simulink model "sampleModel1708_1_sub"  (R2023a)
settings: Solver=VariableStepAuto  StartTime=0.0  StopTime=10.0  RelTol=1e-3
libraries: simulink x4, hdlsllib x3
settings Model: Creator=user1  LastModifiedBy=user1
settings OptimizationCC: BlockReduction=off  ConditionallyExecuteInputs=off

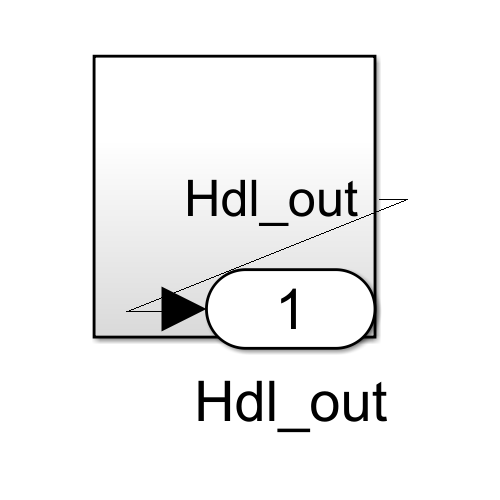
[thumbnail: Simulink's stored preview of the top-level diagram]
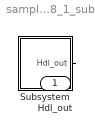
== system sampleModel1708_1_sub ==
  Subsystem : Subsystem
  Hdl_out : Outport  OutDataTypeStr=uint8
  wires:
  Subsystem/1(Hdl_out) -> Hdl_out/1

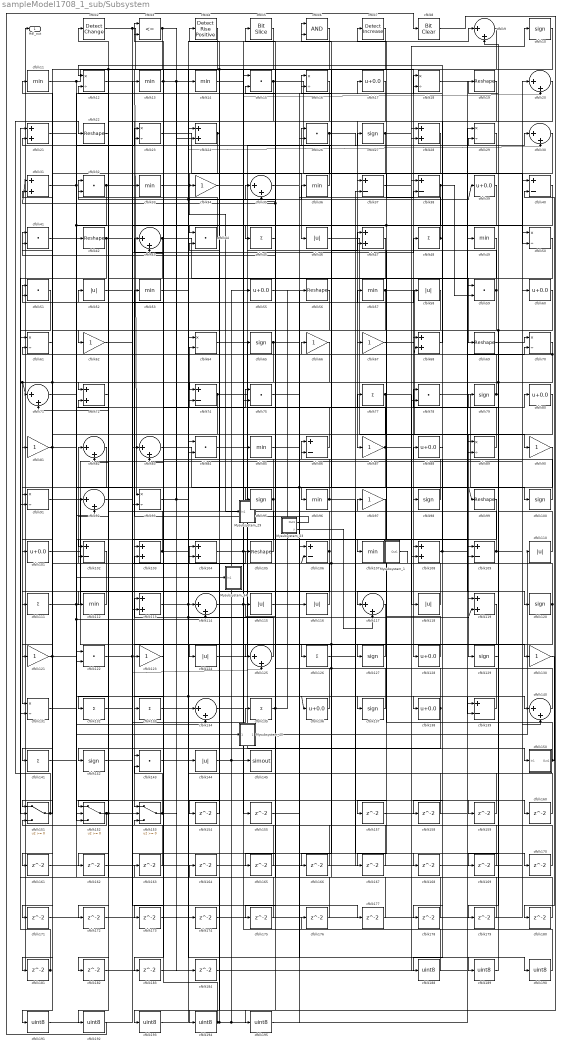
== system sampleModel1708_1_sub/Subsystem ==
  Mysubsystem_1 : Subsystem  TreatAsAtomicUnit=on  RTWFcnName=Mysubsystem_1
      settings: RTWFcnNameOpts=User specified  RTWFileNameOpts=Use function name
  Mysubsystem_23 : Subsystem  TreatAsAtomicUnit=on  RTWFcnName=Mysubsystem_23
      settings: RTWFcnNameOpts=User specified  RTWFileNameOpts=Use function name
  Mysubsystem_29 : Subsystem  TreatAsAtomicUnit=on  RTWFcnName=Mysubsystem_29
      settings: RTWFcnNameOpts=User specified  RTWFileNameOpts=Use function name
  Mysubsystem_34 : Subsystem  TreatAsAtomicUnit=on  RTWFcnName=Mysubsystem_34
      settings: RTWFcnNameOpts=User specified  RTWFileNameOpts=Use function name
  Mysubsystem_40 : Subsystem  TreatAsAtomicUnit=on  RTWFcnName=Mysubsystem_40
      settings: RTWFcnNameOpts=User specified  RTWFileNameOpts=Use function name
  cfblk{10,27,65,79,95,98,100,120,127,129,137,142} (12 alike) : Signum
  cfblk{17,39,55,60,80,88,101,128,136,138} (10 alike) : Bias  Bias=0.0  SaturateOnIntegerOverflow=off
  cfblk{37..38,40,74,86,102,106,109,139} (9 alike) : Sum  Inputs=+-  OutDataTypeStr=uint8
  cfblk{21,24,28,31,47,68,72,103..104,108,113,119} (12 alike) : Sum  OutDataTypeStr=uint8
  cfblk{19,22,42,56,69,99,105} (7 alike) : Reshape
  cfblk{11,13..14,33,36,49,53,57,85,96,107,112} (12 alike) : MinMax  OutDataTypeStr=uint8
  cfblk{46,52,58,110,115..116,118,124,144} (9 alike) : Abs  OutDataTypeStr=uint8  SaturateOnIntegerOverflow=off
  cfblk{45,48,77,111,126,132..133,135,141} (9 alike) : Sum  Inputs=+  OutDataTypeStr=uint8
  cfblk{9,20,30,35,43,71,82..83,92,114,117,125,134,140} (14 alike) : Sum  Inputs=|++  OutDataTypeStr=uint8
  cfblk{12,16,18,23,29,50,61,64,70,89,91,93,131} (13 alike) : Product  Inputs=*/  OutDataTypeStr=uint8  RndMeth=Zero  SaturateOnIntegerOverflow=on
  cfblk{34,62,66..67,81,87,90,97,121,123,130} (11 alike) : Gain  OutDataTypeStr=uint8
  cfblk{15,26,32,41,44,51,59,75,78,84,122,143} (12 alike) : DotProduct  OutDataTypeStr=uint8
  cfblk145 : ToWorkspace  VariableName=simout  SaveFormat=Timeseries  SampleTime=-1
  cfblk150 : Subsystem
      settings: LibrarySourceBlock=|
      | hdlsllib/Ports &
      | Subsystems/Subsystem
  cfblk151 : Switch  OutDataTypeStr=uint8  SaturateOnIntegerOverflow=off  InputSameDT=off
  cfblk152 : Switch  OutDataTypeStr=uint8  SaturateOnIntegerOverflow=off  InputSameDT=off
  cfblk153 : Switch  OutDataTypeStr=uint8  SaturateOnIntegerOverflow=off  InputSameDT=off
  cfblk{154..155,157..184} (30 alike) : Delay  SampleTime=1
  cfblk{188..195} (8 alike) : DataTypeConversion  OutDataTypeStr=uint8  SaturateOnIntegerOverflow=off  RndMeth=Floor
  cfblk2 : simulink/Logic and Bit Operations/Detect Change  vinit=0  OutDataTypeStr=uint8
      settings: LibrarySourceBlock=|
      | hdlsllib/Logic and Bit
      | Operations/Detect
      | Change
  cfblk3 : RelationalOperator  Operator=<=  OutDataTypeStr=boolean  InputSameDT=off
  cfblk4 : hdlsllib/Logic and Bit Operations/Detect Rise Positive  vinit=0  OutDataTypeStr=uint8
  cfblk5 : hdlsllib/Logic and Bit Operations/Bit Slice  lidx=7  ridx=0
  cfblk6 : Logic  AllPortsSameDT=off  OutDataTypeStr=boolean
  cfblk7 : simulink/Logic and Bit Operations/Detect Increase  vinit=0.0  OutDataTypeStr=uint8
      settings: LibrarySourceBlock=|
      | hdlsllib/Logic and Bit
      | Operations/Detect
      | Increase
  cfblk8 : simulink/Logic and Bit Operations/Bit Clear  iBit=0
      settings: LibrarySourceBlock=|
      | hdlsllib/Logic and Bit
      | Operations/Bit Clear
  Hdl_out : Outport  OutDataTypeStr=uint8
  wires:
  cfblk16/1 -> cfblk153/1
  cfblk26/1 -> cfblk29/2, cfblk34/1, Mysubsystem_29/1(In1)
  cfblk11/1 -> cfblk153/2, cfblk128/1
  cfblk17/1 -> cfblk87/1
  cfblk91/1 -> cfblk127/1
  cfblk65/1 -> cfblk30/1, cfblk131/1
  cfblk68/1 -> cfblk12/1
  cfblk57/1 -> cfblk83/2, cfblk90/1
  cfblk121/1 -> cfblk181/1, cfblk74/2
  cfblk10/1 -> cfblk74/1, cfblk93/1
  cfblk84/1 -> cfblk27/1
  cfblk95/1 -> cfblk152/3, cfblk4/1
  cfblk64/1 -> cfblk150/1(In1)
  cfblk106/1 -> cfblk122/2, cfblk43/1
  cfblk52/1 -> cfblk13/1
  cfblk24/1 -> cfblk191/1, cfblk44/1
  cfblk151/1 -> cfblk31/2, cfblk22/1
  cfblk53/1 -> cfblk136/1, cfblk144/1
  cfblk23/1 -> cfblk46/1
  cfblk4/1 -> cfblk123/1
  cfblk9/1 -> cfblk96/1
  cfblk98/1 -> cfblk86/1
  cfblk116/1 -> cfblk82/1
  cfblk124/1 -> cfblk36/1
  cfblk111/1 -> cfblk60/1, Mysubsystem_40/1(In1)
  cfblk105/1 -> cfblk2/1
  cfblk126/1 -> cfblk80/1
  cfblk46/1 -> cfblk129/1
  cfblk78/1 -> cfblk100/1
  cfblk123/1 -> cfblk23/1
  cfblk114/1 -> cfblk6/2, cfblk77/1
  cfblk81/1 -> cfblk41/1, cfblk93/2
  cfblk92/1 -> cfblk48/1
  cfblk29/1 -> cfblk142/1
  cfblk104/1 -> cfblk20/2, cfblk47/1
  cfblk28/1 -> cfblk67/1
  cfblk58/1 -> cfblk107/1
  cfblk137/1 -> cfblk31/1, cfblk32/1
  cfblk3/1 -> cfblk24/2, cfblk162/1, cfblk151/1
  cfblk79/1 -> cfblk9/2, cfblk61/2
  cfblk90/1 -> cfblk141/1
  cfblk56/1 -> cfblk143/1
  cfblk133/1 -> cfblk58/1
  cfblk30/1 -> cfblk68/1
  cfblk83/1 -> cfblk108/1
  cfblk42/1 -> cfblk108/2, cfblk131/2
  cfblk128/1 -> cfblk104/1
  cfblk50/1 -> cfblk103/1
  cfblk6/1 -> cfblk62/1
  cfblk74/1 -> cfblk183/1, cfblk138/1
  cfblk97/1 -> cfblk124/1
  cfblk117/1 -> cfblk166/1, cfblk165/1
  cfblk125/1 -> cfblk113/1
  cfblk70/1 -> cfblk68/2, cfblk169/1, cfblk91/2, cfblk81/1
  cfblk138/1 -> cfblk182/1, cfblk41/2, cfblk6/1
  cfblk39/1 -> cfblk117/1
  cfblk20/1 -> cfblk102/1
  cfblk66/1 -> cfblk101/1, cfblk71/1
  cfblk5/1 -> cfblk84/2
  cfblk127/1 -> cfblk125/1
  cfblk139/1 -> cfblk35/1
  cfblk67/1 -> cfblk98/1
  cfblk102/1 -> cfblk112/1
  cfblk61/1 -> cfblk11/1
  cfblk109/1 -> cfblk44/2, cfblk40/1
  cfblk21/1 -> cfblk50/2, cfblk42/1
  cfblk142/1 -> cfblk135/1
  cfblk48/1 -> cfblk7/1, cfblk18/1
  cfblk15/1 -> cfblk72/1, cfblk50/1
  cfblk69/1 -> cfblk70/1
  cfblk43/1 -> cfblk172/1, cfblk69/1
  cfblk153/1 -> cfblk184/1, cfblk143/2
  cfblk13/1 -> cfblk173/1, cfblk174/1, cfblk45/1
  cfblk112/1 -> cfblk111/1
  cfblk120/1 -> cfblk72/2, cfblk133/1
  cfblk51/1 -> cfblk151/2
  cfblk101/1 -> cfblk119/1
  cfblk113/1 -> cfblk126/1, cfblk9/1
  cfblk75/1 -> cfblk139/2, cfblk99/1
  cfblk87/1 -> cfblk109/2, cfblk121/1, cfblk3/1
  cfblk140/1 -> cfblk26/1
  cfblk150/1(Out1) -> cfblk40/2, cfblk97/1
  cfblk37/1 -> cfblk28/2
  cfblk44/1 -> cfblk12/2
  cfblk93/1 -> cfblk14/1, cfblk30/2, cfblk39/1
  cfblk71/1 -> cfblk92/2
  cfblk143/1 -> cfblk75/1, cfblk119/2
  cfblk77/1 -> cfblk152/1, cfblk118/1
  cfblk59/1 -> cfblk91/1, cfblk16/1
  cfblk99/1 -> cfblk132/1
  cfblk89/1 -> cfblk78/1
  cfblk36/1 -> cfblk21/2
  cfblk103/1 -> cfblk130/1, cfblk71/2
  cfblk135/1 -> cfblk56/1, cfblk115/1
  cfblk107/1 -> cfblk47/2
  cfblk108/1 -> cfblk70/2, cfblk88/1
  cfblk152/1 -> cfblk151/3, cfblk105/1, cfblk52/1
  cfblk100/1 -> cfblk5/1
  cfblk35/1 -> cfblk17/1
  cfblk60/1 -> cfblk95/1, cfblk89/1
  cfblk2/1 -> cfblk177/1, cfblk85/1
  cfblk38/1 -> cfblk59/2, cfblk157/1, cfblk113/2
  cfblk136/1 -> cfblk35/2
  cfblk32/1 -> cfblk152/2, cfblk140/1
  cfblk41/1 -> cfblk134/2
  cfblk31/1 -> cfblk18/2, Mysubsystem_34/1(In1)
  cfblk86/1 -> cfblk64/2
  cfblk118/1 -> cfblk51/1
  cfblk96/1 -> cfblk170/1, cfblk51/2
  cfblk49/1 -> cfblk194/1
  cfblk27/1 -> cfblk10/1, cfblk37/1
  cfblk14/1 -> cfblk109/1
  cfblk72/1 -> cfblk82/2
  cfblk122/1 -> cfblk125/2, cfblk57/1
  cfblk141/1 -> cfblk23/2, cfblk114/2
  cfblk62/1 -> cfblk83/1
  cfblk18/1 -> cfblk120/1
  cfblk110/1 -> cfblk79/1
  cfblk55/1 -> cfblk106/1
  cfblk144/1 -> cfblk65/1, cfblk145/1
  cfblk131/1 -> cfblk137/1
  cfblk115/1 -> cfblk38/2
  cfblk47/1 -> cfblk154/1
  cfblk154/1 -> cfblk104/2
  cfblk34/1 -> cfblk155/1
  cfblk155/1 -> cfblk26/2
  cfblk157/1 -> cfblk89/2
  cfblk119/1 -> cfblk158/1
  cfblk158/1 -> cfblk38/1
  cfblk132/1 -> cfblk159/1
  cfblk159/1 -> cfblk86/2
  cfblk134/1 -> cfblk160/1
  cfblk160/1 -> cfblk84/1
  cfblk82/1 -> cfblk161/1
  cfblk161/1 -> cfblk139/1
  cfblk162/1 -> cfblk37/2
  cfblk163/1 -> cfblk153/3
  cfblk164/1 -> cfblk20/1
  cfblk165/1 -> cfblk92/1
  cfblk166/1 -> cfblk3/2
  cfblk40/1 -> cfblk167/1
  cfblk167/1 -> cfblk43/2
  cfblk12/1 -> cfblk168/1
  cfblk168/1 -> cfblk29/1
  cfblk169/1 -> cfblk24/1
  cfblk170/1 -> cfblk102/2
  cfblk80/1 -> cfblk171/1
  cfblk171/1 -> cfblk64/1
  cfblk172/1 -> cfblk140/2
  cfblk173/1 -> cfblk114/1
  cfblk174/1 -> cfblk75/2
  cfblk45/1 -> cfblk175/1
  cfblk175/1 -> cfblk122/1
  cfblk176/1 -> cfblk15/2
  cfblk177/1 -> cfblk103/2
  cfblk88/1 -> cfblk178/1
  cfblk178/1 -> cfblk61/1
  cfblk129/1 -> cfblk179/1
  cfblk179/1 -> cfblk32/2
  cfblk130/1 -> cfblk180/1
  cfblk180/1 -> cfblk16/2
  cfblk181/1 -> Hdl_out/1, cfblk21/1
  cfblk182/1 -> cfblk28/1
  cfblk183/1 -> cfblk59/1
  cfblk184/1 -> cfblk78/2
  cfblk19/1 -> cfblk188/1
  cfblk188/1 -> cfblk176/1
  cfblk85/1 -> cfblk189/1
  cfblk189/1 -> cfblk19/1
  cfblk33/1 -> cfblk190/1
  cfblk190/1 -> cfblk15/1
  cfblk191/1 -> cfblk33/1
  cfblk22/1 -> cfblk192/1
  cfblk192/1 -> cfblk8/1
  cfblk8/1 -> cfblk193/1
  cfblk193/1 -> cfblk134/1
  cfblk194/1 -> cfblk163/1, cfblk164/1, cfblk116/1, cfblk55/1
  cfblk7/1 -> cfblk195/1
  cfblk195/1 -> cfblk49/1
  Mysubsystem_1/1(Out1) -> cfblk106/2, cfblk66/1
  Mysubsystem_23/1(Out1) -> cfblk53/1
  Mysubsystem_23/2(y) -> cfblk117/2
  Mysubsystem_40/1(Out1) -> cfblk110/1

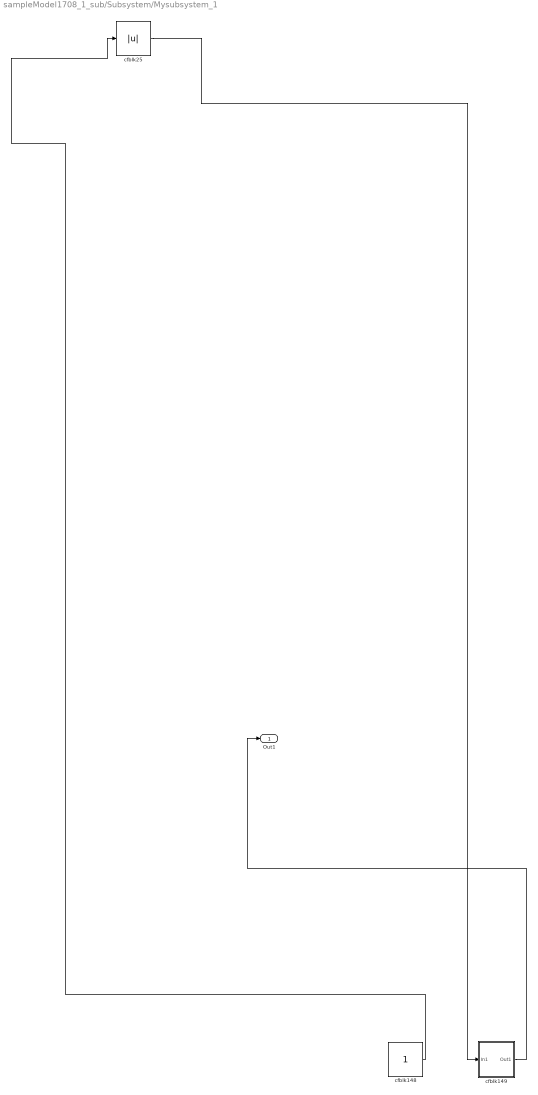
== system sampleModel1708_1_sub/Subsystem/Mysubsystem_1 ==
  cfblk148 : Constant  SampleTime=-1
  cfblk149 : Subsystem
      settings: LibrarySourceBlock=|
      | hdlsllib/Ports &
      | Subsystems/Subsystem
  cfblk25 : Abs  SaturateOnIntegerOverflow=off
  Out1 : Outport
  wires:
  cfblk149/1(Out1) -> Out1/1
  cfblk148/1 -> cfblk25/1
  cfblk25/1 -> cfblk149/1(In1)

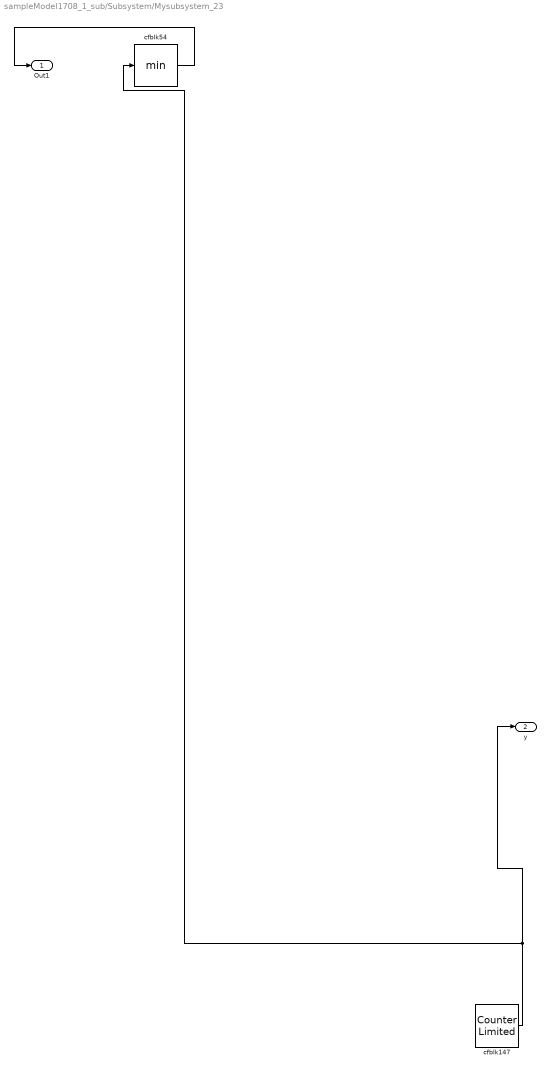
== system sampleModel1708_1_sub/Subsystem/Mysubsystem_23 ==
  cfblk147 : hdlsllib/Sources/Counter Limited  uplimit=7  tsamp=-1
  cfblk54 : MinMax
  Out1 : Outport
  y : Outport  Port=2
  wires:
  cfblk54/1 -> Out1/1
  cfblk147/1 -> cfblk54/1, y/1

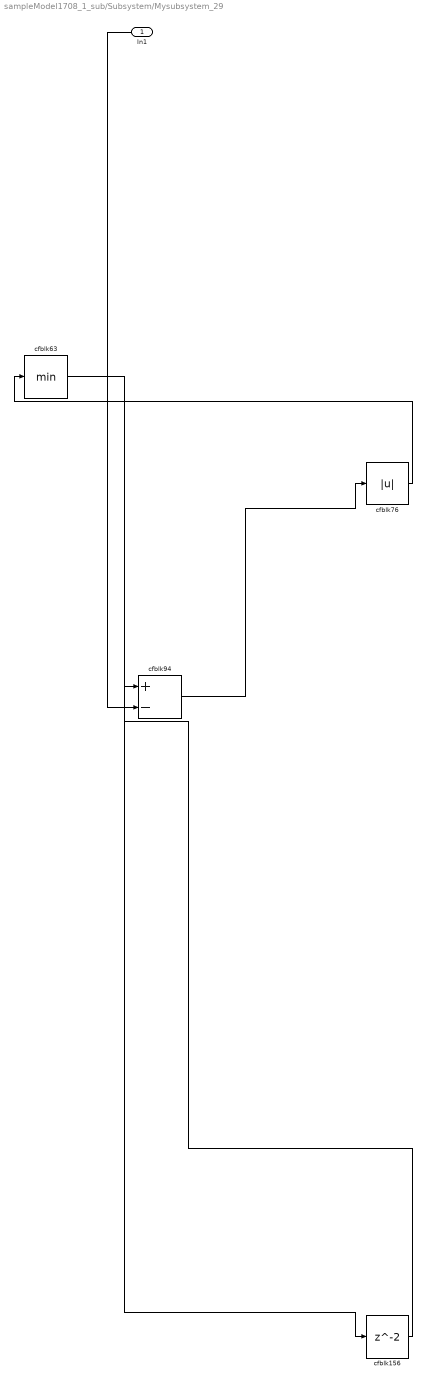
== system sampleModel1708_1_sub/Subsystem/Mysubsystem_29 ==
  In1 : Inport
  cfblk156 : Delay  SampleTime=1
  cfblk63 : MinMax
  cfblk76 : Abs  SaturateOnIntegerOverflow=off
  cfblk94 : Sum  Inputs=+-
  wires:
  cfblk94/1 -> cfblk76/1
  cfblk76/1 -> cfblk63/1
  In1/1 -> cfblk94/2
  cfblk156/1 -> cfblk94/1
  cfblk63/1 -> cfblk156/1

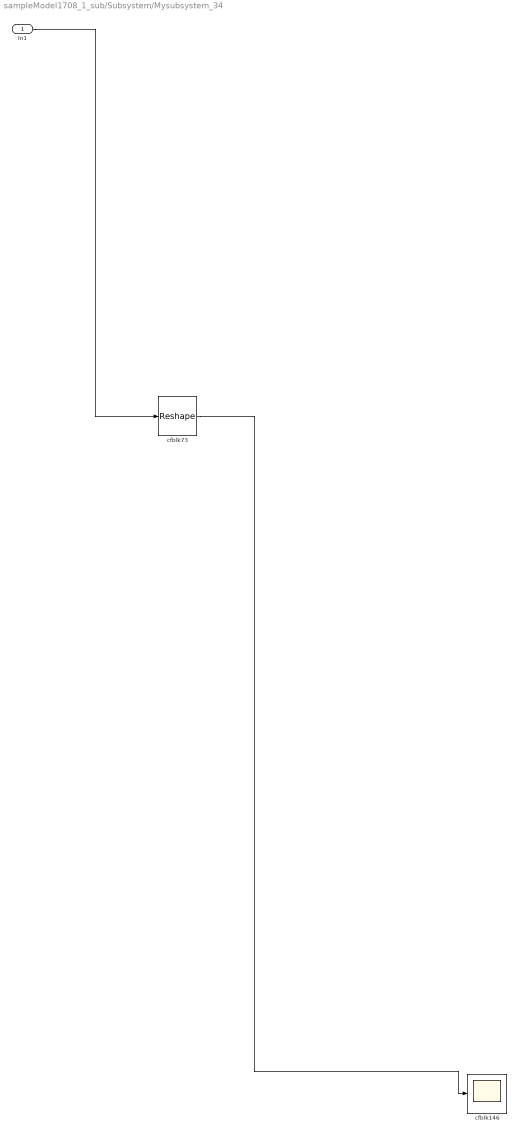
== system sampleModel1708_1_sub/Subsystem/Mysubsystem_34 ==
  In1 : Inport
  cfblk146 : Scope
  cfblk73 : Reshape
  wires:
  In1/1 -> cfblk73/1
  cfblk73/1 -> cfblk146/1

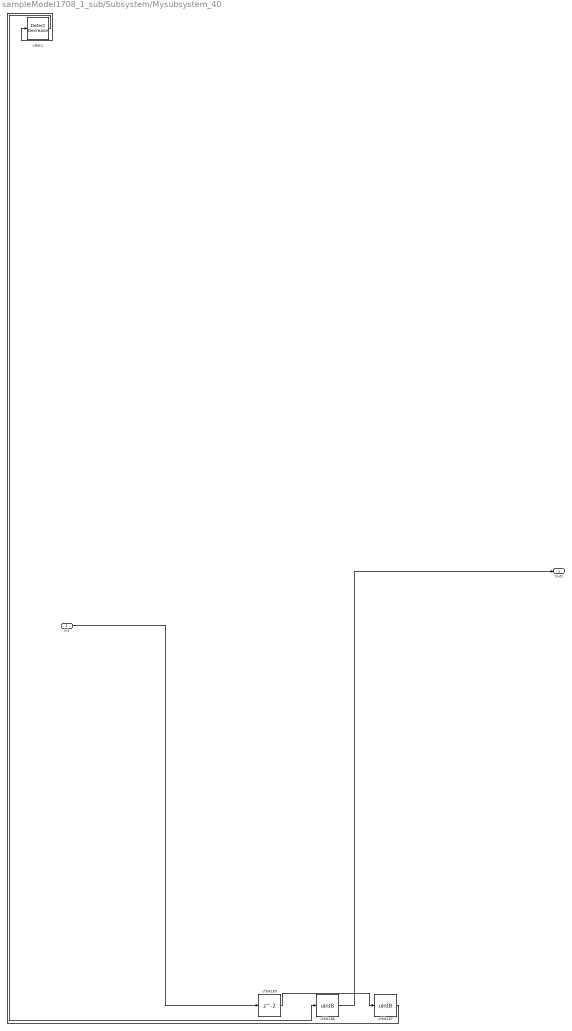
== system sampleModel1708_1_sub/Subsystem/Mysubsystem_40 ==
  In1 : Inport
  cfblk1 : simulink/Logic and Bit Operations/Detect Decrease  vinit=0.0  OutDataTypeStr=boolean
      settings: LibrarySourceBlock=|
      | hdlsllib/Logic and Bit
      | Operations/Detect
      | Decrease
  cfblk185 : Delay  SampleTime=1
  cfblk186 : DataTypeConversion  OutDataTypeStr=uint8  SaturateOnIntegerOverflow=off  RndMeth=Floor
  cfblk187 : DataTypeConversion  OutDataTypeStr=uint8  SaturateOnIntegerOverflow=off  RndMeth=Floor
  Out1 : Outport
  wires:
  In1/1 -> cfblk185/1
  cfblk186/1 -> Out1/1
  cfblk1/1 -> cfblk186/1
  cfblk187/1 -> cfblk1/1
  cfblk185/1 -> cfblk187/1

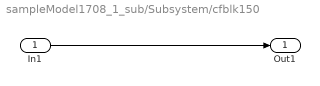
== system sampleModel1708_1_sub/Subsystem/cfblk150 ==
  In1 : Inport
  Out1 : Outport
  wires:
  In1/1 -> Out1/1

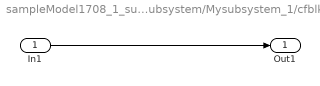
== system sampleModel1708_1_sub/Subsystem/Mysubsystem_1/cfblk149 ==
  In1 : Inport
  Out1 : Outport
  wires:
  In1/1 -> Out1/1
